simulink model "ellip_fit"  (R2023a)
settings: Solver=VariableStepAuto  StartTime=0.0  StopTime=1.0  RelTol=1e-3
values from neighbouring files (symbols this model uses):
  x = 5 + 4*cos(t) + rand(size(t))    [ellipLinReg2.m]    (also in presim_runmefirst.m = data(:,1))
  y = 8 + 2*sin(t) + rand(size(t))    [ellipLinReg2.m]    (also in presim_runmefirst.m = data(:,2))
settings Model: Creator=DWAMAI  LastModifiedBy=DWAMAI

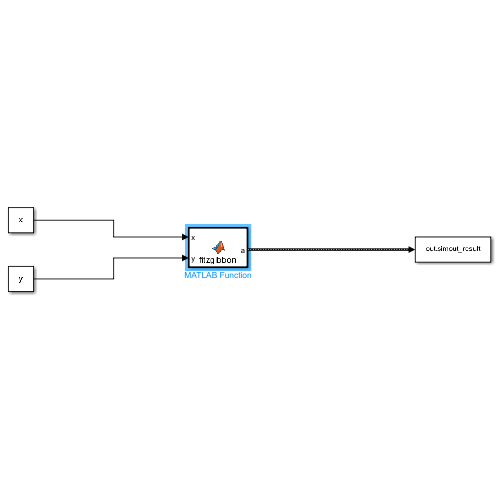
[thumbnail: Simulink's stored preview of the top-level diagram]
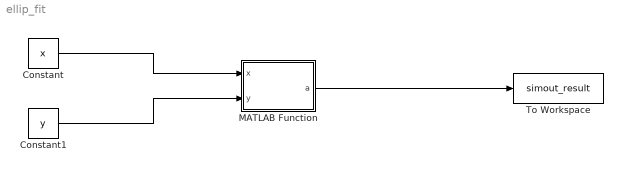
== system ellip_fit ==
  Constant : Constant  Value=x
  Constant1 : Constant  Value=y
  MATLAB Function : MATLAB Function  TreatAsAtomicUnit=on
  To Workspace : ToWorkspace  VariableName=simout_result  SaveFormat=Structure  SampleTime=1
      settings: Decimation=99
  wires:
  Constant/1 -> MATLAB Function/1(x)
  MATLAB Function/1(a) -> To Workspace/1
  Constant1/1 -> MATLAB Function/2(y)

== matlab function ellip_fit/MATLAB Function ==
  settings: updateMethod=DISCRETE  sampleTime=1
  data: x input; a output size=[6,1]; y input
function a = fitzgibbon(x,y)

D1 = [x .^ 2, x .* y, y .^ 2 ];
D2 = [x,y, ones(size(x))];

S1 = D1' * D1;
S2 = D1' * D2;
S3 = D2' * D2;

T = - inv(S3) * S2';

M = S1 + S2 * T;
M = [M(3, :) ./ 2; - M(2, :); M(1, :) ./ 2];

[evec, eval] = eig(M);

cond = 4 * evec(1, :) .* evec(3, :) - evec(2, :) .^ 2;

%a1 = evec(:, find(cond > 0));
a1 = evec(:, cond > 0);

a = [a1; T * a1];

end
